simulink model "main"  (R2025b)
settings: Solver=ode4  StartTime=0.0  StopTime=60  FixedStep=Ts_inner  RelTol=1e-3
undefined symbols (not defined in the file): Ts_gcs
libraries: aerolibutil x4, sldrtlib x1
settings Model: DataDictionary=project.sldd  Creator=Nick  LastModifiedBy=Nick
settings SolverCC: AutoInsertRateTranBlk=on

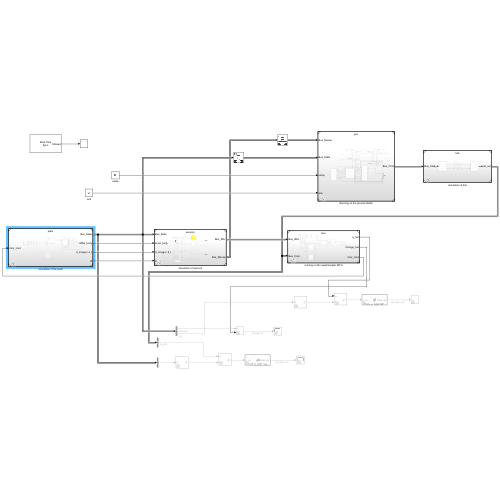
[thumbnail: Simulink's stored preview of the top-level diagram]
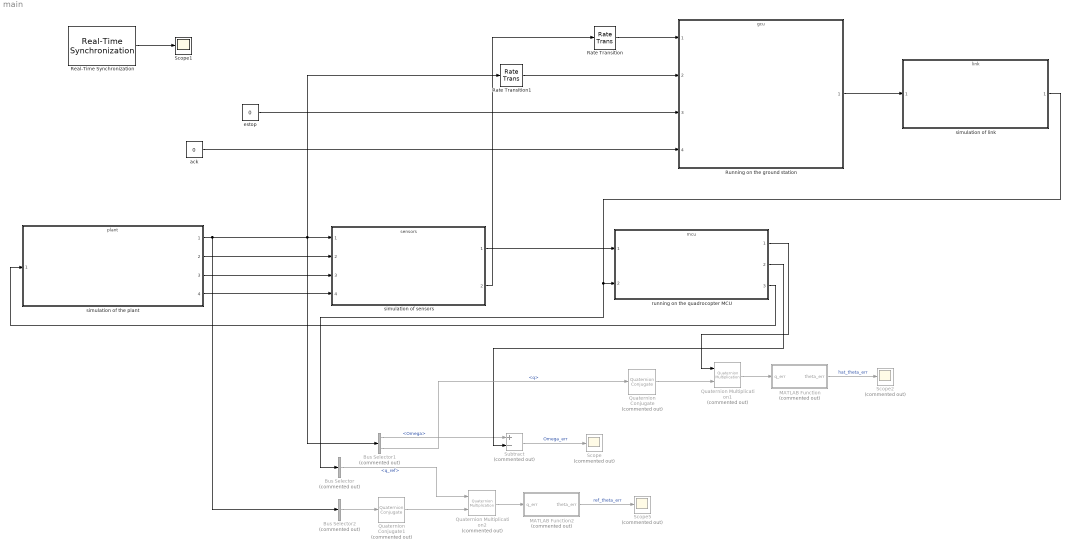
== system main ==
  Bus Selector : BusSelector  Commented=on  OutputSignals=q_ref
  Bus Selector1 : BusSelector  Commented=on  OutputSignals=Omega,q
  Bus Selector2 : BusSelector  Commented=on  OutputSignals=q  OutputAsBus=on
  MATLAB Function : MATLAB Function  Commented=on  TreatAsAtomicUnit=on
  MATLAB Function2 : MATLAB Function  Commented=on  TreatAsAtomicUnit=on
  Quaternion Conjugate : aerolibutil/Quaternion Conjugate  Commented=on
  Quaternion Conjugate1 : aerolibutil/Quaternion Conjugate  Commented=on
  Quaternion Multiplication1 : aerolibutil/Quaternion Multiplication  Commented=on
  Quaternion Multiplication2 : aerolibutil/Quaternion Multiplication  Commented=on
  Rate Transition : RateTransition  OutPortSampleTime=Ts_gcs
  Rate Transition1 : RateTransition  OutPortSampleTime=Ts_gcs
  Real-Time Synchronization : sldrtlib/Real-Time Synchronization  SampleTime=Ts_gcs  MaxMissedTicks=inf  ShowMissedTicks=on  YieldWhenWaiting=off
  Running on the ground station : ModelReference  ModelNameDialog=gcu.slx  SimulationMode=Normal  ModelReferenceVersion=1.286
  Scope : Scope  Commented=on
      settings: ActiveDisplayYMinimum=-1  ActiveDisplayYMaximum=1
  Scope1 : Scope
      settings: ActiveDisplayYMinimum=-1  ActiveDisplayYMaximum=1
  Scope2 : Scope  Commented=on
      settings: ActiveDisplayYMinimum=-0.084122920988905683  ActiveDisplayYMaximum=0.78039338720264007  DataLoggingVariableName=ScopeData2
  Scope5 : Scope  Commented=on
      settings: ActiveDisplayYMinimum=-0.013956380673274989  ActiveDisplayYMaximum=0.12560742605947492  DataLoggingVariableName=ScopeData5
  Subtract : Sum  Commented=on  Inputs=+-
  ack : Constant  Value=0  OutDataTypeStr=boolean
  estop : Constant  Value=0  OutDataTypeStr=uint8
  running on the quadrocopter MCU : ModelReference  ModelNameDialog=mcu.slx  SimulationMode=Normal  ModelReferenceVersion=1.228
  simulation of link : ModelReference  ModelNameDialog=link.slx  SimulationMode=Normal  ModelReferenceVersion=1.112
  simulation of sensors : ModelReference  ModelNameDialog=sensors.slx  SimulationMode=Normal  ModelReferenceVersion=1.80
  simulation of the plant : ModelReference  ModelNameDialog=plant.slx  SimulationMode=Normal  ModelReferenceVersion=1.181
  wires:
  simulation of the plant/1 -> Bus Selector2/1, Rate Transition1/1, Bus Selector1/1, simulation of sensors/1
  simulation of the plant/2 -> simulation of sensors/2
  simulation of the plant/3 -> simulation of sensors/3
  simulation of the plant/4 -> simulation of sensors/4
  simulation of sensors/1 -> running on the quadrocopter MCU/1
  simulation of sensors/2 -> Rate Transition/1
  Quaternion Conjugate/1 -> Quaternion Multiplication1/2
  MATLAB Function/1(theta_err) -> Scope2/1  "hat_theta_err"
  Quaternion Multiplication1/1 -> MATLAB Function/1(q_err)
  running on the quadrocopter MCU/1 -> Quaternion Multiplication1/1
  Bus Selector1/1 -> Subtract/1  "<Omega>"
  running on the quadrocopter MCU/2 -> Subtract/2
  Subtract/1 -> Scope/1  "Omega_err"
  Bus Selector1/2 -> Quaternion Conjugate/1  "<q>"
  running on the quadrocopter MCU/3 -> simulation of the plant/1
  Bus Selector2/1 -> Quaternion Conjugate1/1
  Quaternion Multiplication2/1 -> MATLAB Function2/1(q_err)
  MATLAB Function2/1(theta_err) -> Scope5/1  "ref_theta_err"
  Quaternion Conjugate1/1 -> Quaternion Multiplication2/2
  Running on the ground station/1 -> simulation of link/1
  Rate Transition/1 -> Running on the ground station/1
  Rate Transition1/1 -> Running on the ground station/2
  Bus Selector/1 -> Quaternion Multiplication2/1  "<q_ref>"
  simulation of link/1 -> Bus Selector/1, running on the quadrocopter MCU/2
  Real-Time Synchronization/1 -> Scope1/1
  estop/1 -> Running on the ground station/3
  ack/1 -> Running on the ground station/4

== matlab function main/MATLAB Function2 ==
  data: q_err input; theta_err output
function theta_err = quat_2_rotAngle(q_err)   %#codegen
    theta_err = 2*atan2(norm(q_err(2:4)), abs(q_err(1)));
end

== matlab function main/MATLAB Function ==
  data: q_err input; theta_err output
function theta_err = quat_2_rotAngle(q_err)   
%#codegen
    theta_err = 2*atan2(norm(q_err(2:4)), abs(q_err(1)));
end
